simulink model "controller_verified0ne_for_boost"  (R2024b)
settings: Solver=VariableStepAuto  StartTime=0.0  StopTime=0.5  RelTol=1e-6
values from neighbouring files (symbols this model uses):
  beta = Rb/(Ra+Rb)    (= 0.25)    [code_with_nonlinearity.m]
  Tm = 1    [code_with_nonlinearity.m]
undefined symbols (not defined in the file or in its folder): den, Mv_den, mv_num, num, tp_den, tp_num, Z0_den, Z0_num
libraries: simulink x2
settings Model: Creator=S SURYA  LastModifiedBy=S SURYA

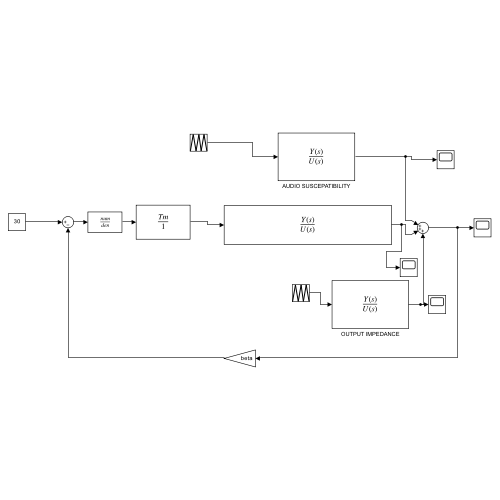
[thumbnail: Simulink's stored preview of the top-level diagram]
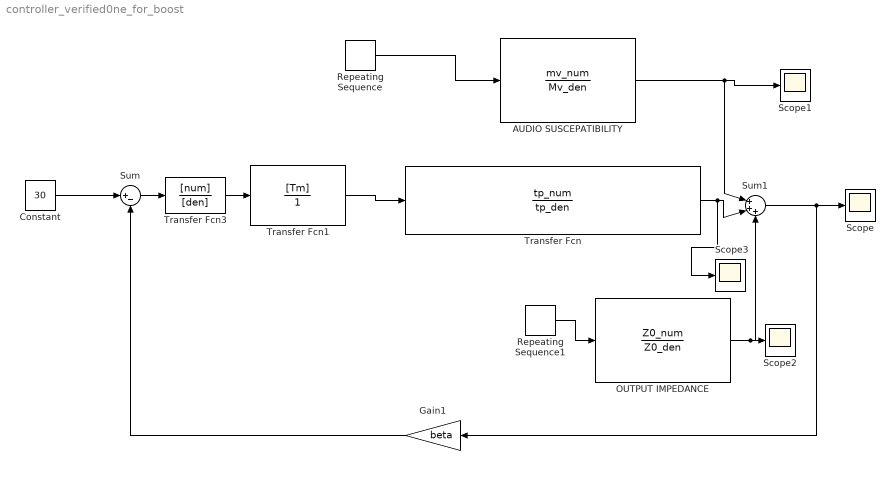
== system controller_verified0ne_for_boost ==
  AUDIO SUSCEPATIBILITY : TransferFcn  Numerator=mv_num  Denominator=Mv_den
  Constant : Constant  Value=30
  Gain1 : Gain  Gain=beta
  OUTPUT IMPEDANCE : TransferFcn  Numerator=Z0_num  Denominator=Z0_den
  Repeating Sequence : simulink/Sources/Repeating Sequence  rep_seq_t=[0 5e-6 10e-6]  rep_seq_y=[0 1 0]
  Repeating Sequence1 : simulink/Sources/Repeating Sequence  rep_seq_t=[0 5e-6 10e-6]  rep_seq_y=[0 1 0]
  Scope{,1..3} (4 alike) : Scope
  Sum : Sum  Inputs=|+-
  Sum1 : Sum  Inputs=|+++
  Transfer Fcn : TransferFcn  Numerator=tp_num  Denominator=tp_den
  Transfer Fcn1 : TransferFcn  Numerator=[Tm]  Denominator=[1]
  Transfer Fcn3 : TransferFcn  Numerator=[num]  Denominator=[den]
  wires:
  Transfer Fcn1/1 -> Transfer Fcn/1
  Transfer Fcn3/1 -> Transfer Fcn1/1
  Gain1/1 -> Sum/2
  Sum/1 -> Transfer Fcn3/1
  Constant/1 -> Sum/1
  Sum1/1 -> Gain1/1, Scope/1
  AUDIO SUSCEPATIBILITY/1 -> Sum1/1, Scope1/1
  Transfer Fcn/1 -> Scope3/1, Sum1/2
  OUTPUT IMPEDANCE/1 -> Sum1/3, Scope2/1
  Repeating Sequence/1 -> AUDIO SUSCEPATIBILITY/1
  Repeating Sequence1/1 -> OUTPUT IMPEDANCE/1
